simulink library "libsb2sl"  (Simulink 7.3)
settings: Solver=ode45  SolverMode=SingleTasking  StartTime=0.0  StopTime=10.0  RelTol=1e-3
PostLoadFcn:
  | setsysloc libsb2sl
undefined symbols (not defined in the file): A, Ac, Ad, B, Bc, Bd, C, Cc, Cd, code, const, D, data, Dc, Dd, DiscIntNeverNeededParam, gain, info, k, m, map, no, stat, X0, xd, xi
libraries: simulink3 x17, simulink x5, libsb2sl x3
(part 2 of 3)

== system libsb2sl/DYN/DResetIntegrator ==
  1stOrder : Subsystem  mask(DYN-Palette){IMODE=Forward Euler, RMODE=Single edge, K=1, X0=0, TS=0.1}
      mask prompts: IMODE "Integrator Method:"; RMODE "External Reset:"; K "Output Gains:"; X0 "Initial Conditions:"; TS "Sampling Time:"
      mask help: Nth order integration of an input with resettable states.
      mask init:
      | operator={'rising','either'};
      | method={'ForwardEuler';'BackwardEuler';'Trapezoidal'};
      | set_param([gcb  '/Integrator'],'ExternalReset',operator{RMODE},'IntegratorMethod',method{IMODE});
      | [x,y]=sblibico('1stOrderReset','disc');
      mask StyleString: popup(Forward Euler|Backward Euler|Trapezoidal),popup(Single edge|Double edge),edit,edit,edit
      mask Display: plot(0,0,1,1,x,y)
  1stOrder1 : Subsystem  mask(DYN-Palette){IMODE=Forward Euler, RMODE=Single edge, X0=0, TS=0.1}
      mask prompts: IMODE "Integrator Method:"; RMODE "External Reset:"; X0 "Initial Conditions:"; TS "Sampling Time:"
      mask help: Nth order integration of an input with resettable states.
      mask init:
      | operator={'rising','either'};
      | method={'ForwardEuler';'BackwardEuler';'Trapezoidal'};
      | set_param([gcb  '/Integrator'],'ExternalReset',operator{RMODE},'IntegratorMethod',method{IMODE});
      | [x,y]=sblibico('1stOrder1Reset','disc');
      mask StyleString: popup(Forward Euler|Backward Euler|Trapezoidal),popup(Single edge|Double edge),edit,edit
      mask Display: plot(0,0,1,1,x,y)
  NthOrder : Subsystem  mask(DYN-Palette){IMODE=Forward Euler, N=1, RMODE=Single edge, NR=1, K=1, X0=0, TS=0.1}
      mask prompts: IMODE "Integrator Method:"; N "Order of Integration:"; RMODE "External Reset:"; NR "Highest Order of Resettable State:"; K "Output Gains:"; X0 "Initial Conditions:"; TS "Sampling Time:"
      mask help: Nth order integration of an input with resettable states.
      mask init:
      | no=length(K);
      | [stateMap,resetMap]=sblibdrv('Integrator',N,no,NR);
      | operator={'rising','either'};
      | method={'ForwardEuler';'BackwardEuler';'Trapezoidal'};
      | set_param([gcb  '/Integrator'],'ExternalReset',operator{RMODE},'IntegratorMethod',method{IMODE});
      | [x,y]=sblibico('nthOrderReset','disc');
      mask StyleString: popup(Forward Euler|Backward Euler|Trapezoidal),edit,popup(Single edge|Double edge),edit,edit,edit,edit
      mask Display: plot(0,0,1,1,x,y)
  NthOrder1 : Subsystem  mask(DYN-Palette){IMODE=Forward Euler, N=1, RMODE=Single edge, NR=1, X0=0, TS=0.1}
      mask prompts: IMODE "Integrator Method:"; N "Order of Integration:"; RMODE "External Reset:"; NR "Highest Order of Resettable State:"; X0 "Initial Conditions:"; TS "Sampling Time:"
      mask help: Nth order integration of an input with resettable states.
      mask init:
      | no=length(X0)/N;
      | [stateMap,resetMap]=sblibdrv('Integrator',N,no,NR);
      | operator={'rising','either'};
      | method={'ForwardEuler';'BackwardEuler';'Trapezoidal'};
      | set_param([gcb  '/Integrator'],'ExternalReset',operator{RMODE},'IntegratorMethod',method{IMODE});
      | [x,y]=sblibico('nthOrder1Reset','disc');
      mask StyleString: popup(Forward Euler|Backward Euler|Trapezoidal),edit,popup(Single edge|Double edge),edit,edit,edit
      mask Display: plot(0,0,1,1,x,y)

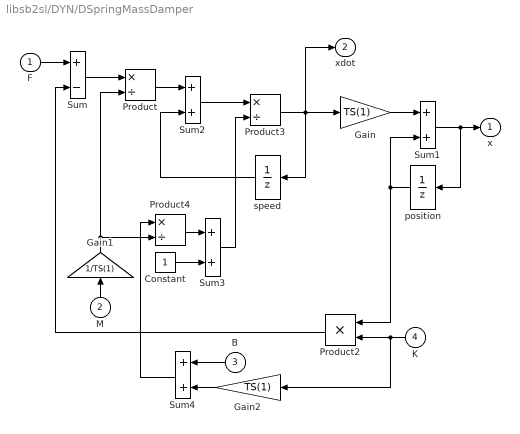
== system libsb2sl/DYN/DSpringMassDamper ==
  F : Inport  SampleTime=TS  OutDataType=sfix(16)  OutScaling=2^0
  M : Inport  Port=2  SampleTime=TS  OutDataType=sfix(16)  OutScaling=2^0
  B : Inport  Port=3  SampleTime=TS  OutDataType=sfix(16)  OutScaling=2^0
  K : Inport  Port=4  SampleTime=TS  OutDataType=sfix(16)  OutScaling=2^0
  Constant : Constant  OutDataType=sfix(16)  OutScaling=2^0
  Gain : Gain  Gain=TS(1)  ParameterDataType=sfix(16)  ParameterScaling=2^0  OutDataType=sfix(16)  OutScaling=2^0  SaturateOnIntegerOverflow=on  OutDataTypeStr=Inherit: Same as input  ParamDataTypeStr=Inherit: Same as input
  Gain1 : Gain  Gain=1/TS(1)  ParameterDataType=sfix(16)  ParameterScaling=2^0  OutDataType=sfix(16)  OutScaling=2^0  SaturateOnIntegerOverflow=on  OutDataTypeStr=Inherit: Same as input  ParamDataTypeStr=Inherit: Same as input
  Gain2 : Gain  Gain=TS(1)  ParameterDataType=sfix(16)  ParameterScaling=2^0  OutDataType=sfix(16)  OutScaling=2^0  SaturateOnIntegerOverflow=on  OutDataTypeStr=Inherit: Same as input  ParamDataTypeStr=Inherit: Same as input
  Product : Product  Inputs=*/  OutDataType=sfix(16)  OutScaling=2^0  SaturateOnIntegerOverflow=on  RndMeth=Zero  InputSameDT=on  OutDataTypeStr=Inherit: Same as first input
  Product2 : Product  OutDataType=sfix(16)  OutScaling=2^0  SaturateOnIntegerOverflow=on  RndMeth=Zero  InputSameDT=on  OutDataTypeStr=Inherit: Same as first input
  Product3 : Product  Inputs=*/  OutDataType=sfix(16)  OutScaling=2^0  SaturateOnIntegerOverflow=on  RndMeth=Zero  InputSameDT=on  OutDataTypeStr=Inherit: Same as first input
  Product4 : Product  Inputs=*/  OutDataType=sfix(16)  OutScaling=2^0  SaturateOnIntegerOverflow=on  RndMeth=Zero  InputSameDT=on  OutDataTypeStr=Inherit: Same as first input
  Sum : Sum  Inputs=+-  OutDataType=sfix(16)  OutScaling=2^0  SaturateOnIntegerOverflow=on  InputSameDT=on  OutDataTypeStr=Inherit: Same as first input
  Sum{1..4} (4 alike) : Sum  OutDataType=sfix(16)  OutScaling=2^0  SaturateOnIntegerOverflow=on  InputSameDT=on  OutDataTypeStr=Inherit: Same as first input
  position : UnitDelay  X0=X0(1)  SampleTime=TS
  speed : UnitDelay  X0=X0(2)  SampleTime=TS
  x : Outport  OutDataType=sfix(16)  OutScaling=2^0  InitialOutput=X0(1)
  xdot : Outport  Port=2  OutDataType=sfix(16)  OutScaling=2^0  InitialOutput=X0(2)
  wires:
  Sum4/1 -> Product4/1
  Gain2/1 -> Sum4/2
  B/1 -> Sum4/1
  K/1 -> Gain2/1, Product2/2
  Gain1/1 -> Product4/2, Product/2
  M/1 -> Gain1/1
  position/1 -> Product2/1, Sum1/2
  Sum3/1 -> Product3/2
  Product2/1 -> Sum/2
  Sum1/1 -> position/1, x/1
  Gain/1 -> Sum1/1
  Product3/1 -> xdot/1, Gain/1, speed/1
  Product4/1 -> Sum3/1
  Constant/1 -> Sum3/2
  speed/1 -> Sum2/2
  Sum2/1 -> Product3/1
  Product/1 -> Sum2/1
  Sum/1 -> Product/1
  F/1 -> Sum/1

== system libsb2sl/DYN/DStateSpace ==
  u : Inport  OutDataType=sfix(16)  OutScaling=2^0
  StateSpace : DiscreteStateSpace  A=A  B=B  C=C  D=D  X0=X0  SampleTime=TS
  y : Outport  OutDataType=sfix(16)  OutScaling=2^0
  wires:
  u/1 -> StateSpace/1
  StateSpace/1 -> y/1

== system libsb2sl/DYN/DTimeDelay ==
  u : Inport  SampleTime=TS  OutDataType=sfix(16)  OutScaling=2^0
  Demux : Demux  Outputs=[no no (k+1)*no]
  Mux : Mux  Inputs=[no (k+1)*no]
  Selector : Selector  InputPortWidth=(k+2)*no  IndexOptions=Index vector (dialog)  Indices=[k*no+1:(k+2)*no 1:(k+1)*no]  OutputSizes=1
  Sum : Sum  Inputs=+|+  OutDataType=sfix(16)  OutScaling=2^0  SaturateOnIntegerOverflow=on  InputSameDT=on  OutDataTypeStr=Inherit: Same as first input
  Unit Delay : UnitDelay  X0=X0  SampleTime=TS
  m : Gain  Gain=1-m  ParameterDataType=sfix(16)  ParameterScaling=2^0  OutDataType=sfix(16)  OutScaling=2^0  SaturateOnIntegerOverflow=on  OutDataTypeStr=Inherit: Same as input  ParamDataTypeStr=Inherit: Same as input
  m1 : Gain  Gain=m  ParameterDataType=sfix(16)  ParameterScaling=2^0  OutDataType=sfix(16)  OutScaling=2^0  SaturateOnIntegerOverflow=on  OutDataTypeStr=Inherit: Same as input  ParamDataTypeStr=Inherit: Same as input
  y : Outport  OutDataType=sfix(16)  OutScaling=2^0
  wires:
  u/1 -> Mux/1
  Unit Delay/1 -> Mux/2
  Mux/1 -> Selector/1
  Sum/1 -> y/1
  m1/1 -> Sum/2
  m/1 -> Sum/1
  Demux/2 -> m1/1
  Demux/1 -> m/1
  Demux/3 -> Unit Delay/1
  Selector/1 -> Demux/1

== system libsb2sl/LOG/Decoder ==
  u : Inport  OutDataType=sfix(16)  OutScaling=2^0
  decoder : S-Function  FunctionName=sbdecoder  Parameters=BPI,MIN,MAX  EnableBusSupport=off
  y : Outport  OutDataType=sfix(16)  OutScaling=2^0
  wires:
  u/1 -> decoder/1
  decoder/1 -> y/1

== system libsb2sl/LOG/EQV ==
  u1 : Inport  OutDataType=sfix(16)  OutScaling=2^0
  u2 : Inport  Port=2  OutDataType=sfix(16)  OutScaling=2^0
  EQV : Logic  Operator=NOT  Inputs=1
  NEQV : Logic  Operator=XOR
  bool1 : RelationalOperator  Operator=>  InputSameDT=on
  bool2 : RelationalOperator  Operator=>  InputSameDT=on
  zero : Constant  Value=0  OutDataType=sfix(16)  OutScaling=2^0  OutDataTypeStr=Inherit: Inherit via back propagation
  y : Outport  OutDataType=sfix(16)  OutScaling=2^0
  wires:
  bool1/1 -> NEQV/1
  bool2/1 -> NEQV/2
  u1/1 -> bool1/1
  u2/1 -> bool2/1
  zero/1 -> bool2/2, bool1/2
  NEQV/1 -> EQV/1
  EQV/1 -> y/1

== system libsb2sl/LOG/Encoder ==
  u : Inport  OutDataType=sfix(16)  OutScaling=2^0
  encoder : S-Function  FunctionName=sbencoder  Parameters=BPO,MIN,MAX  EnableBusSupport=off
  y : Outport  OutDataType=sfix(16)  OutScaling=2^0
  wires:
  u/1 -> encoder/1
  encoder/1 -> y/1

== system libsb2sl/LOG/GainScheduler ==
  s : Inport  OutDataType=sfix(16)  OutScaling=2^0
  u : Inport  Port=2  OutDataType=sfix(16)  OutScaling=2^0
  sbgainsched : S-Function  FunctionName=sbgainsched  Parameters=IND,GAIN  EnableBusSupport=off
  y : Outport  OutDataType=sfix(16)  OutScaling=2^0
  wires:
  s/1 -> sbgainsched/1
  sbgainsched/1 -> y/1
  u/1 -> sbgainsched/2

== system libsb2sl/LOG/LogExpression ==
  u : Inport  OutDataType=sfix(16)  OutScaling=2^0
  sblogexp : S-Function  FunctionName=sblogexp  Parameters=code,stat,data,info,P0,TS  EnableBusSupport=off
  y : Outport  OutDataType=sfix(16)  OutScaling=2^0
  wires:
  u/1 -> sblogexp/1
  sblogexp/1 -> y/1

== system libsb2sl/LOG/NEQV ==
  u1 : Inport  OutDataType=sfix(16)  OutScaling=2^0
  u2 : Inport  Port=2  OutDataType=sfix(16)  OutScaling=2^0
  NEQV : Logic  Operator=XOR
  bool1 : RelationalOperator  Operator=>  InputSameDT=on
  bool2 : RelationalOperator  Operator=>  InputSameDT=on
  zero : Constant  Value=0  OutDataType=sfix(16)  OutScaling=2^0  OutDataTypeStr=Inherit: Inherit via back propagation
  y : Outport  OutDataType=sfix(16)  OutScaling=2^0
  wires:
  bool1/1 -> NEQV/1
  bool2/1 -> NEQV/2
  u1/1 -> bool1/1
  NEQV/1 -> y/1
  u2/1 -> bool2/1
  zero/1 -> bool1/2, bool2/2

== system libsb2sl/LOG/NOT ==
  u1 : Inport  OutDataType=sfix(16)  OutScaling=2^0
  bool1 : RelationalOperator  Operator=>  InputSameDT=on
  logic : Logic  Operator=NOT
  zero : Constant  Value=0  OutDataType=sfix(16)  OutScaling=2^0  OutDataTypeStr=Inherit: Inherit via back propagation
  y : Outport  OutDataType=sfix(16)  OutScaling=2^0
  wires:
  bool1/1 -> logic/1
  u1/1 -> bool1/1
  logic/1 -> y/1
  zero/1 -> bool1/2

== system libsb2sl/LOG/ShiftRegister ==
  u : Inport  SampleTime=TS  OutDataType=sfix(16)  OutScaling=2^0
  sbshiftreg : S-Function  FunctionName=sbshiftreg  Parameters=NX,NY,X0,TS  EnableBusSupport=off
  y : Outport  OutDataType=sfix(16)  OutScaling=2^0
  wires:
  u/1 -> sbshiftreg/1
  sbshiftreg/1 -> y/1

== system libsb2sl/LOG/Switch ==
  u1 : Inport  OutDataType=sfix(16)  OutScaling=2^0
  u2 : Inport  Port=2  OutDataType=sfix(16)  OutScaling=2^0
  u3 : Inport  Port=3  OutDataType=sfix(16)  OutScaling=2^0
  Switch : Switch  Criteria=u2 > Threshold  SaturateOnIntegerOverflow=on  InputSameDT=on
  y : Outport  OutDataType=sfix(16)  OutScaling=2^0
  wires:
  Switch/1 -> y/1
  u2/1 -> Switch/1
  u3/1 -> Switch/3
  u1/1 -> Switch/2

== system libsb2sl/MAT/Constant ==
  Constant : Constant  Value=constantValue  OutDataType=sfix(16)  OutScaling=2^0
  Y : Outport  OutDataType=sfix(16)  OutScaling=2^0
  wires:
  Constant/1 -> Y/1

== system libsb2sl/MAT/LeftMultiply ==
  A : Inport  OutDataType=sfix(16)  OutScaling=2^0
  Matrix Gain : Gain  Gain=G  Multiplication=Matrix(u*K)  ParameterDataType=sfix(16)  ParameterScaling=2^0  OutDataType=sfix(16)  OutScaling=2^0  SaturateOnIntegerOverflow=on  OutDataTypeStr=Inherit: Same as input  ParamDataTypeStr=Inherit: Same as input
  Y2y : simulink/Math Operations/Reshape  OutputDimensionality=1-D array  OutputDimensions=[1,1]
  a2A : simulink/Math Operations/Reshape  OutputDimensionality=Customize  OutputDimensions=[nACols,nARows]
  Y : Outport  OutDataType=sfix(16)  OutScaling=2^0
  wires:
  A/1 -> a2A/1
  Y2y/1 -> Y/1
  Matrix Gain/1 -> Y2y/1
  a2A/1 -> Matrix Gain/1

== system libsb2sl/MAT/MatLeftDivide ==
  A : Inport  OutDataType=sfix(16)  OutScaling=2^0
  B : Inport  Port=2  OutDataType=sfix(16)  OutScaling=2^0
  Product : Product  Inputs=*/  Multiplication=Matrix(*)  OutDataType=sfix(16)  OutScaling=2^0  SaturateOnIntegerOverflow=on  RndMeth=Zero  InputSameDT=on  OutDataTypeStr=Inherit: Same as first input
  Y2y : simulink3/Signals & Systems/Reshape  OutputDimensionality=1-D array  OutputDimensions=[1,1]
  a2A : simulink3/Signals & Systems/Reshape  OutputDimensionality=Customize  OutputDimensions=[nACols,nARows]
  b2B : simulink3/Signals & Systems/Reshape  OutputDimensionality=Customize  OutputDimensions=[nBCols,nBRows]
  Y : Outport  OutDataType=sfix(16)  OutScaling=2^0
  wires:
  Product/1 -> Y2y/1
  B/1 -> b2B/1
  Y2y/1 -> Y/1
  A/1 -> a2A/1
  b2B/1 -> Product/1
  a2A/1 -> Product/2

== system libsb2sl/MAT/MatRightDivide ==
  A : Inport  OutDataType=sfix(16)  OutScaling=2^0
  B : Inport  Port=2  OutDataType=sfix(16)  OutScaling=2^0
  Product : Product  Inputs=/*  Multiplication=Matrix(*)  OutDataType=sfix(16)  OutScaling=2^0  SaturateOnIntegerOverflow=on  RndMeth=Zero  InputSameDT=on  OutDataTypeStr=Inherit: Same as first input
  Y2y : simulink3/Signals & Systems/Reshape  OutputDimensionality=1-D array  OutputDimensions=[1,1]
  a2A : simulink3/Signals & Systems/Reshape  OutputDimensionality=Customize  OutputDimensions=[nACols,nARows]
  b2B : simulink3/Signals & Systems/Reshape  OutputDimensionality=Customize  OutputDimensions=[nBCols,nBRows]
  Y : Outport  OutDataType=sfix(16)  OutScaling=2^0
  wires:
  b2B/1 -> Product/2
  a2A/1 -> Product/1
  Product/1 -> Y2y/1
  A/1 -> a2A/1
  Y2y/1 -> Y/1
  B/1 -> b2B/1

== system libsb2sl/MAT/MatrixInverse ==
  A : Inport  OutDataType=sfix(16)  OutScaling=2^0
  Product : Product  Inputs=/  Multiplication=Matrix(*)  OutDataType=sfix(16)  OutScaling=2^0  SaturateOnIntegerOverflow=on  RndMeth=Zero  InputSameDT=on  OutDataTypeStr=Inherit: Same as first input
  Y2y : simulink3/Signals & Systems/Reshape  OutputDimensionality=1-D array  OutputDimensions=[1,1]
  a2A : simulink3/Signals & Systems/Reshape  OutputDimensionality=Customize  OutputDimensions=[nACols,nARows]
  Y : Outport  OutDataType=sfix(16)  OutScaling=2^0
  wires:
  A/1 -> a2A/1
  Y2y/1 -> Y/1
  a2A/1 -> Product/1
  Product/1 -> Y2y/1

== system libsb2sl/MAT/MatrixMultiply ==
  A : Inport  OutDataType=sfix(16)  OutScaling=2^0
  B : Inport  Port=2  OutDataType=sfix(16)  OutScaling=2^0
  Product : Product  Inputs=**  Multiplication=Matrix(*)  OutDataType=sfix(16)  OutScaling=2^0  SaturateOnIntegerOverflow=on  RndMeth=Zero  InputSameDT=on  OutDataTypeStr=Inherit: Same as first input
  Y2y : simulink3/Signals & Systems/Reshape  OutputDimensionality=1-D array  OutputDimensions=[1,1]
  a2A : simulink3/Signals & Systems/Reshape  OutputDimensionality=Customize  OutputDimensions=[nACols,nARows]
  b2B : simulink3/Signals & Systems/Reshape  OutputDimensionality=Customize  OutputDimensions=[nBCols,nBRows]
  Y : Outport  OutDataType=sfix(16)  OutScaling=2^0
  wires:
  a2A/1 -> Product/2
  b2B/1 -> Product/1
  B/1 -> b2B/1
  Y2y/1 -> Y/1
  A/1 -> a2A/1
  Product/1 -> Y2y/1

== system libsb2sl/MAT/MatrixTranspose ==
  A : Inport  OutDataType=sfix(16)  OutScaling=2^0
  Selector : Selector  InputPortWidth=nARows*nACols  IndexOptions=Index vector (dialog)  Indices=mapIndices(:)  OutputSizes=1
  Y : Outport  OutDataType=sfix(16)  OutScaling=2^0
  wires:
  Selector/1 -> Y/1
  A/1 -> Selector/1

== system libsb2sl/MAT/RightMultiply ==
  A : Inport  OutDataType=sfix(16)  OutScaling=2^0
  Matrix Gain : Gain  Gain=G  Multiplication=Matrix(K*u)  ParameterDataType=sfix(16)  ParameterScaling=2^0  OutDataType=sfix(16)  OutScaling=2^0  SaturateOnIntegerOverflow=on  OutDataTypeStr=Inherit: Same as input  ParamDataTypeStr=Inherit: Same as input
  Y2y : Reshape
  a2A : Reshape  OutputDimensionality=Customize  OutputDimensions=[nACols,nARows]
  Y : Outport  OutDataType=sfix(16)  OutScaling=2^0
  wires:
  a2A/1 -> Matrix Gain/1
  Matrix Gain/1 -> Y2y/1
  Y2y/1 -> Y/1
  A/1 -> a2A/1

== system libsb2sl/NTP/BiCubicInterp ==
  note: Swap inputs to accommodate
      | Row-major 2-D tables in
      | SystemBuild
  u1 : Inport  OutDataType=sfix(16)  OutScaling=2^0
  u2 : Inport  Port=2  OutDataType=sfix(16)  OutScaling=2^0
  Look-Up Table (n-D) : simulink3/Functions & Tables/Look-Up Table (n-D)  numDimsPopupSelect=2  bp1=in2BrkPoints  bp2=in1BrkPoints  explicitNumDims=2  searchMode=Binary Search  cacheBpFlag=on  vectorInputFlag=off  tableData=outBrkPoints  interpMethod=Cubic Spline  extrapMethod=None - Clip  rangeErrorMode=Error
  y : Outport  OutDataType=sfix(16)  OutScaling=2^0
  wires:
  u1/1 -> Look-Up Table (n-D)/2
  u2/1 -> Look-Up Table (n-D)/1
  Look-Up Table (n-D)/1 -> y/1

== system libsb2sl/NTP/BiLinearInterp ==
  note: Swap inputs to accommodate
      | Row-major 2-D tables in
      | SystemBuild
  u1 : Inport  OutDataType=sfix(16)  OutScaling=2^0
  u2 : Inport  Port=2  OutDataType=sfix(16)  OutScaling=2^0
  Look-Up Table (n-D) : simulink3/Functions & Tables/Look-Up Table (n-D)  numDimsPopupSelect=2  bp1=in2BrkPoints  bp2=in1BrkPoints  explicitNumDims=2  searchMode=Binary Search  cacheBpFlag=on  vectorInputFlag=off  tableData=outBrkPoints  interpMethod=Linear  extrapMethod=Linear  rangeErrorMode=None
  y : Outport  OutDataType=sfix(16)  OutScaling=2^0
  wires:
  u2/1 -> Look-Up Table (n-D)/1
  u1/1 -> Look-Up Table (n-D)/2
  Look-Up Table (n-D)/1 -> y/1

== system libsb2sl/NTP/ConstantInterp ==
  u : Inport  OutDataType=sfix(16)  OutScaling=2^0
  Look-Up Table (n-D) : simulink3/Functions & Tables/Look-Up Table (n-D)  numDimsPopupSelect=1  bp1=in1BrkPoints  explicitNumDims=1  searchMode=Binary Search  cacheBpFlag=on  vectorInputFlag=on  tableData=outBrkPoints  interpMethod=None - Flat  extrapMethod=None - Clip  rangeErrorMode=None
  y : Outport  OutDataType=sfix(16)  OutScaling=2^0
  wires:
  Look-Up Table (n-D)/1 -> y/1
  u/1 -> Look-Up Table (n-D)/1

== system libsb2sl/NTP/CubicInterp ==
  u : Inport  OutDataType=sfix(16)  OutScaling=2^0
  Look-Up Table (n-D) : simulink3/Functions & Tables/Look-Up Table (n-D)  numDimsPopupSelect=1  bp1=in1BrkPoints  explicitNumDims=1  searchMode=Binary Search  cacheBpFlag=on  vectorInputFlag=on  tableData=outBrkPoints  interpMethod=Cubic Spline  extrapMethod=Cubic Spline  rangeErrorMode=None
  y : Outport  OutDataType=sfix(16)  OutScaling=2^0
  wires:
  u/1 -> Look-Up Table (n-D)/1
  Look-Up Table (n-D)/1 -> y/1

== system libsb2sl/NTP/LinearInterp ==
  u : Inport  OutDataType=sfix(16)  OutScaling=2^0
  Look-Up Table (n-D) : simulink3/Functions & Tables/Look-Up Table (n-D)  numDimsPopupSelect=1  bp1=in1BrkPoints  explicitNumDims=1  searchMode=Binary Search  cacheBpFlag=on  vectorInputFlag=on  tableData=outBrkPoints  interpMethod=Linear  extrapMethod=Linear  rangeErrorMode=None
  y : Outport  OutDataType=sfix(16)  OutScaling=2^0
  wires:
  u/1 -> Look-Up Table (n-D)/1
  Look-Up Table (n-D)/1 -> y/1

== system libsb2sl/NTP/MultiLinearInterp ==
  u : Inport  OutDataType=sfix(16)  OutScaling=2^0
  multilinear interp : simulink/Lookup Tables/Lookup Table (n-D)  numDimsPopupSelect=More...  bp1=in1BrkPoints  bp2=in2BrkPoints  bp3=in3BrkPoints  bp4=in4BrkPoints  bpcell={in5BrkPoints,in6BrkPoints,in7BrkPoints,in8BrkPoints}  explicitNumDims=NINP+1  searchMode=Linear Search  cacheBpFlag=on  vectorInputFlag=on  tableData=tableData  interpMethod=Linear  extrapMethod=Linear  rangeErrorMode=None
  y : Outport  OutDataType=sfix(16)  OutScaling=2^0
  wires:
  multilinear interp/1 -> y/1
  u/1 -> multilinear interp/1

== system libsb2sl/PEL/Constant**u ==
  u : Inport  OutDataType=sfix(16)  OutScaling=2^0
  Constant : Constant  Value=CONST  OutDataType=sfix(16)  OutScaling=2^0
  Power : Math  Operator=pow  OutDataType=sfix(16)  OutScaling=2^0  SaturateOnIntegerOverflow=on
  y : Outport  OutDataType=sfix(16)  OutScaling=2^0
  wires:
  Power/1 -> y/1
  Constant/1 -> Power/1
  u/1 -> Power/2

== system libsb2sl/PEL/SignedSqrt ==
  u : Inport  OutDataType=sfix(16)  OutScaling=2^0
  Abs : Abs  SaturateOnIntegerOverflow=on
  Math Function : Math  Operator=sqrt  OutDataType=sfix(16)  OutScaling=2^0  SaturateOnIntegerOverflow=on
  Product : Product  OutDataType=sfix(16)  OutScaling=2^0  SaturateOnIntegerOverflow=on  RndMeth=Zero  InputSameDT=on  OutDataTypeStr=Inherit: Same as first input
  Sign : Signum
  y : Outport  OutDataType=sfix(16)  OutScaling=2^0
  wires:
  Math Function/1 -> Product/1
  Sign/1 -> Product/2
  Abs/1 -> Math Function/1
  Product/1 -> y/1
  u/1 -> Abs/1, Sign/1

== system libsb2sl/PEL/u**Constant ==
  u : Inport  OutDataType=sfix(16)  OutScaling=2^0
  Constant : Constant  Value=CONST  OutDataType=sfix(16)  OutScaling=2^0
  Power : Math  Operator=pow  OutDataType=sfix(16)  OutScaling=2^0  SaturateOnIntegerOverflow=on
  y : Outport  OutDataType=sfix(16)  OutScaling=2^0
  wires:
  Power/1 -> y/1
  u/1 -> Power/1
  Constant/1 -> Power/2

== system libsb2sl/PWL/Preload ==
  u : Inport  OutDataType=sfix(16)  OutScaling=2^0
  Constant : Constant  Value=preload  OutDataType=sfix(16)  OutScaling=2^0
  Constant1 : Constant  Value=-preload  OutDataType=sfix(16)  OutScaling=2^0
  Sum : Sum  OutDataType=sfix(16)  OutScaling=2^0  SaturateOnIntegerOverflow=on  InputSameDT=on  OutDataTypeStr=Inherit: Same as first input
  Switch : Switch  SaturateOnIntegerOverflow=on  InputSameDT=on
  slope : Gain  Gain=slope  ParameterDataType=sfix(16)  ParameterScaling=2^0  OutDataType=sfix(16)  OutScaling=2^0  SaturateOnIntegerOverflow=on  OutDataTypeStr=Inherit: Same as input  ParamDataTypeStr=Inherit: Same as input
  y : Outport  OutDataType=sfix(16)  OutScaling=2^0
  wires:
  slope/1 -> Sum/2
  Switch/1 -> Sum/1
  u/1 -> Switch/2, slope/1
  Sum/1 -> y/1
  Constant/1 -> Switch/1
  Constant1/1 -> Switch/3

== system libsb2sl/PWL/Quantization ==
  u : Inport  OutDataType=sfix(16)  OutScaling=2^0
  Resolution : Constant  Value=RES  OutDataType=sfix(16)  OutScaling=2^0
  Type : Rounding  Operator=round
  div : Product  Inputs=*/  OutDataType=sfix(16)  OutScaling=2^0  SaturateOnIntegerOverflow=on  RndMeth=Zero  InputSameDT=on  OutDataTypeStr=Inherit: Same as first input
  mul : Product  OutDataType=sfix(16)  OutScaling=2^0  SaturateOnIntegerOverflow=on  RndMeth=Zero  InputSameDT=on  OutDataTypeStr=Inherit: Same as first input
  y : Outport  OutDataType=sfix(16)  OutScaling=2^0
  wires:
  div/1 -> Type/1
  Type/1 -> mul/1
  Resolution/1 -> div/2, mul/2
  u/1 -> div/1
  mul/1 -> y/1

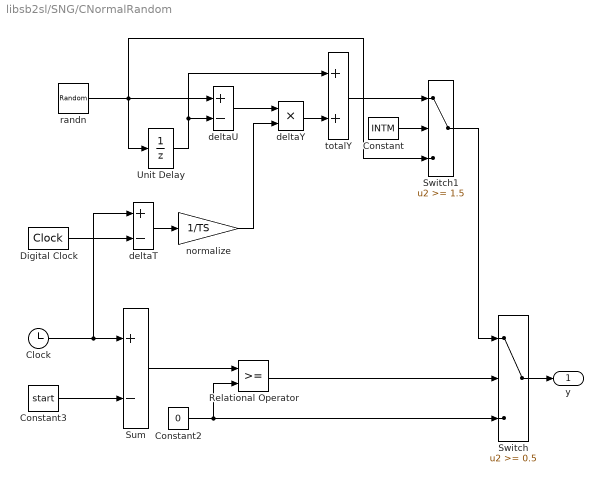
== system libsb2sl/SNG/CNormalRandom ==
  Clock : Clock
      settings: Decimation=10
  Constant : Constant  Value=INTM  OutDataType=sfix(16)  OutScaling=2^0
  Constant2 : Constant  Value=0  OutDataType=sfix(16)  OutScaling=2^0
  Constant3 : Constant  Value=start  OutDataType=sfix(16)  OutScaling=2^0
  Digital Clock : DigitalClock  SampleTime=TS
  Relational Operator : RelationalOperator  InputSameDT=on
  Sum : Sum  Inputs=+-  OutDataType=sfix(16)  OutScaling=2^0  SaturateOnIntegerOverflow=on  InputSameDT=on  OutDataTypeStr=Inherit: Same as first input
  Switch : Switch  Threshold=0.5  SaturateOnIntegerOverflow=on  InputSameDT=on
  Switch1 : Switch  Threshold=1.5  SaturateOnIntegerOverflow=on  InputSameDT=on
  Unit Delay : UnitDelay  SampleTime=TS
  deltaT : Sum  Inputs=+-  OutDataType=sfix(16)  OutScaling=2^0  SaturateOnIntegerOverflow=on  InputSameDT=on  OutDataTypeStr=Inherit: Same as first input
  deltaU : Sum  Inputs=+-  OutDataType=sfix(16)  OutScaling=2^0  SaturateOnIntegerOverflow=on  InputSameDT=on  OutDataTypeStr=Inherit: Same as first input
  deltaY : Product  OutDataType=sfix(16)  OutScaling=2^0  SaturateOnIntegerOverflow=on  RndMeth=Zero  InputSameDT=on  OutDataTypeStr=Inherit: Same as first input
  normalize : Gain  Gain=1/TS  ParameterDataType=sfix(16)  ParameterScaling=2^0  OutDataType=sfix(16)  OutScaling=2^0  SaturateOnIntegerOverflow=on  OutDataTypeStr=Inherit: Same as input  ParamDataTypeStr=Inherit: Same as input
  randn : RandomNumber  Mean=MEAN  Variance=STD.^2  Seed=SEED  SampleTime=TS
  totalY : Sum  OutDataType=sfix(16)  OutScaling=2^0  SaturateOnIntegerOverflow=on  InputSameDT=on  OutDataTypeStr=Inherit: Same as first input
  y : Outport  OutDataType=sfix(16)  OutScaling=2^0
  wires:
  Clock/1 -> deltaT/1, Sum/1
  Switch/1 -> y/1
  Switch1/1 -> Switch/1
  Constant2/1 -> Switch/3, Relational Operator/2
  Relational Operator/1 -> Switch/2
  Sum/1 -> Relational Operator/1
  Constant3/1 -> Sum/2
  randn/1 -> deltaU/1, Unit Delay/1, Switch1/3
  Constant/1 -> Switch1/2
  totalY/1 -> Switch1/1
  Unit Delay/1 -> deltaU/2, totalY/1
  deltaY/1 -> totalY/2
  normalize/1 -> deltaY/2
  deltaU/1 -> deltaY/1
  deltaT/1 -> normalize/1
  Digital Clock/1 -> deltaT/2

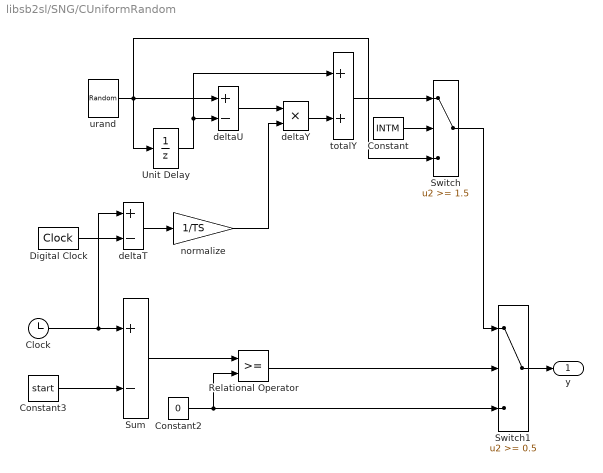
== system libsb2sl/SNG/CUniformRandom ==
  Clock : Clock
      settings: Decimation=10
  Constant : Constant  Value=INTM  OutDataType=sfix(16)  OutScaling=2^0
  Constant2 : Constant  Value=0  OutDataType=sfix(16)  OutScaling=2^0
  Constant3 : Constant  Value=start  OutDataType=sfix(16)  OutScaling=2^0
  Digital Clock : DigitalClock  SampleTime=TS
  Relational Operator : RelationalOperator  InputSameDT=on
  Sum : Sum  Inputs=+-  OutDataType=sfix(16)  OutScaling=2^0  SaturateOnIntegerOverflow=on  InputSameDT=on  OutDataTypeStr=Inherit: Same as first input
  Switch : Switch  Threshold=1.5  SaturateOnIntegerOverflow=on  InputSameDT=on
  Switch1 : Switch  Threshold=0.5  SaturateOnIntegerOverflow=on  InputSameDT=on
  Unit Delay : UnitDelay  SampleTime=TS
  deltaT : Sum  Inputs=+-  OutDataType=sfix(16)  OutScaling=2^0  SaturateOnIntegerOverflow=on  InputSameDT=on  OutDataTypeStr=Inherit: Same as first input
  deltaU : Sum  Inputs=+-  OutDataType=sfix(16)  OutScaling=2^0  SaturateOnIntegerOverflow=on  InputSameDT=on  OutDataTypeStr=Inherit: Same as first input
  deltaY : Product  OutDataType=sfix(16)  OutScaling=2^0  SaturateOnIntegerOverflow=on  RndMeth=Zero  InputSameDT=on  OutDataTypeStr=Inherit: Same as first input
  normalize : Gain  Gain=1/TS  ParameterDataType=sfix(16)  ParameterScaling=2^0  OutDataType=sfix(16)  OutScaling=2^0  SaturateOnIntegerOverflow=on  OutDataTypeStr=Inherit: Same as input  ParamDataTypeStr=Inherit: Same as input
  totalY : Sum  OutDataType=sfix(16)  OutScaling=2^0  SaturateOnIntegerOverflow=on  InputSameDT=on  OutDataTypeStr=Inherit: Same as first input
  urand : UniformRandomNumber  Minimum=MIN  Maximum=MAX  Seed=SEED  SampleTime=TS
  y : Outport  OutDataType=sfix(16)  OutScaling=2^0
  wires:
  Constant2/1 -> Relational Operator/2, Switch1/3
  Relational Operator/1 -> Switch1/2
  Sum/1 -> Relational Operator/1
  Constant3/1 -> Sum/2
  Switch1/1 -> y/1
  Constant/1 -> Switch/2
  totalY/1 -> Switch/1
  Unit Delay/1 -> totalY/1, deltaU/2
  deltaY/1 -> totalY/2
  normalize/1 -> deltaY/2
  deltaU/1 -> deltaY/1
  deltaT/1 -> normalize/1
  Digital Clock/1 -> deltaT/2
  urand/1 -> Switch/3, Unit Delay/1, deltaU/1
  Switch/1 -> Switch1/1
  Clock/1 -> Sum/1, deltaT/1

== system libsb2sl/SNG/DNormalRandom ==
  Clock : Clock
      settings: Decimation=10
  Constant2 : Constant  Value=0  OutDataType=sfix(16)  OutScaling=2^0
  Constant3 : Constant  Value=start  OutDataType=sfix(16)  OutScaling=2^0
  Relational Operator : RelationalOperator  InputSameDT=on
  Sum : Sum  Inputs=+-  OutDataType=sfix(16)  OutScaling=2^0  SaturateOnIntegerOverflow=on  InputSameDT=on  OutDataTypeStr=Inherit: Same as first input
  Switch : Switch  Threshold=0.5  SaturateOnIntegerOverflow=on  InputSameDT=on
  randn : RandomNumber  Mean=MEAN  Variance=STD.^2  Seed=SEED  SampleTime=TS
  y : Outport  OutDataType=sfix(16)  OutScaling=2^0
  wires:
  randn/1 -> Switch/1
  Clock/1 -> Sum/1
  Constant3/1 -> Sum/2
  Sum/1 -> Relational Operator/1
  Relational Operator/1 -> Switch/2
  Constant2/1 -> Relational Operator/2, Switch/3
  Switch/1 -> y/1

== system libsb2sl/SNG/DUniformRandom ==
  Clock : Clock
      settings: Decimation=10
  Constant2 : Constant  Value=0  OutDataType=sfix(16)  OutScaling=2^0
  Constant3 : Constant  Value=start  OutDataType=sfix(16)  OutScaling=2^0
  Relational Operator : RelationalOperator  InputSameDT=on
  Sum : Sum  Inputs=+-  OutDataType=sfix(16)  OutScaling=2^0  SaturateOnIntegerOverflow=on  InputSameDT=on  OutDataTypeStr=Inherit: Same as first input
  Switch : Switch  Threshold=0.5  SaturateOnIntegerOverflow=on  InputSameDT=on
  urand : UniformRandomNumber  Minimum=MIN  Maximum=MAX  Seed=SEED  SampleTime=TS
  y : Outport  OutDataType=sfix(16)  OutScaling=2^0
  wires:
  Clock/1 -> Sum/1
  Constant3/1 -> Sum/2
  Sum/1 -> Relational Operator/1
  Relational Operator/1 -> Switch/2
  Constant2/1 -> Switch/3, Relational Operator/2
  Switch/1 -> y/1
  urand/1 -> Switch/1

== system libsb2sl/SNG/GenWaveform ==
  Clock : Clock
      settings: Decimation=10
  Constant1 : Constant  Value=period  OutDataType=sfix(16)  OutScaling=2^0
  Constant2 : Constant  Value=0  OutDataType=sfix(16)  OutScaling=2^0
  Constant3 : Constant  Value=start  OutDataType=sfix(16)  OutScaling=2^0
  LinearInterp : libsb2sl/NTP/LinearInterp  SystemSampleTime=-1  in1BrkPoints=in1BrkPoints  outBrkPoints=outBrkPoints
  Math Function : Math  Operator=rem  OutDataType=sfix(16)  OutScaling=2^0  SaturateOnIntegerOverflow=on
  Sum : Sum  Inputs=+-  OutDataType=sfix(16)  OutScaling=2^0  SaturateOnIntegerOverflow=on  InputSameDT=on  OutDataTypeStr=Inherit: Same as first input
  Switch : Switch  SaturateOnIntegerOverflow=on  InputSameDT=on
  y : Outport  OutDataType=sfix(16)  OutScaling=2^0
  wires:
  Clock/1 -> Sum/1
  Switch/1 -> y/1
  Sum/1 -> Math Function/1, Switch/2
  Constant3/1 -> Sum/2
  Constant2/1 -> Switch/3
  Constant1/1 -> Math Function/2
  Math Function/1 -> LinearInterp/1
  LinearInterp/1 -> Switch/1

== system libsb2sl/SNG/LimRamp ==
  Compare To Zero : simulink/Logic and Bit Operations/Compare To Zero  SystemSampleTime=-1  relop=~=  LogicOutDataTypeMode=boolean  ZeroCross=off
  Constant5 : Constant  Value=SAT  OutDataType=sfix(16)  OutScaling=2^0
  Constant6 : Constant  Value=RATE  OutDataType=sfix(16)  OutScaling=2^0
  Data Type Conversion : DataTypeConversion  OutDataType=fixdt(1, 16)  OutScaling=2^0
  Product : Product  OutDataType=sfix(16)  OutScaling=2^0  SaturateOnIntegerOverflow=on  RndMeth=Zero  InputSameDT=on  OutDataTypeStr=Inherit: Same as first input
  Product1 : Product  OutDataType=sfix(16)  OutScaling=2^0  SaturateOnIntegerOverflow=on  RndMeth=Zero  InputSameDT=on  OutDataTypeStr=Inherit: Same as first input
  Ramp : simulink/Sources/Ramp  SystemSampleTime=-1  slope=RATE  start=start  X0=0
  Sum1 : Sum  Inputs=-+  OutDataType=sfix(16)  OutScaling=2^0  SaturateOnIntegerOverflow=on  InputSameDT=on  OutDataTypeStr=Inherit: Same as first input
  Switch1 : Switch  SaturateOnIntegerOverflow=on  InputSameDT=on
  y : Outport  OutDataType=sfix(16)  OutScaling=2^0
  wires:
  Data Type Conversion/1 -> Product1/2
  Product1/1 -> Switch1/3
  Compare To Zero/1 -> Data Type Conversion/1
  Ramp/1 -> Compare To Zero/1, Switch1/1, Sum1/1
  Constant6/1 -> Product/2
  Sum1/1 -> Product/1
  Constant5/1 -> Product1/1, Sum1/2
  Switch1/1 -> y/1
  Product/1 -> Switch1/2

== system libsb2sl/SNG/PulseTrain ==
  Pulse Generator1 : DiscretePulseGenerator  PulseType=Time based  Amplitude=A  Period=1./F  PulseWidth=PW.*F*100  PhaseDelay=start  SampleTime=1
  y : Outport  OutDataType=sfix(16)  OutScaling=2^0
  wires:
  Pulse Generator1/1 -> y/1

== system libsb2sl/SNG/SinusoidGen ==
  Clock : Clock
      settings: Decimation=10
  Constant2 : Constant  Value=0  OutDataType=sfix(16)  OutScaling=2^0
  Constant3 : Constant  Value=start  OutDataType=sfix(16)  OutScaling=2^0
  Relational Operator : RelationalOperator  InputSameDT=on
  Sine Wave : Sin  TimeSource=Use external signal  Amplitude=A  Bias=0  Frequency=2*pi*F  Phase=pi*PHI/180  Samples=10  SampleTime=0  Offset=0
  Sum : Sum  Inputs=+-  OutDataType=sfix(16)  OutScaling=2^0  SaturateOnIntegerOverflow=on  InputSameDT=on  OutDataTypeStr=Inherit: Same as first input
  Switch : Switch  Threshold=0.5  SaturateOnIntegerOverflow=on  InputSameDT=on
  y : Outport  OutDataType=sfix(16)  OutScaling=2^0
  wires:
  Switch/1 -> y/1
  Sine Wave/1 -> Switch/1
  Constant2/1 -> Switch/3, Relational Operator/2
  Relational Operator/1 -> Switch/2
  Constant3/1 -> Sum/2
  Clock/1 -> Sum/1
  Sum/1 -> Sine Wave/1, Relational Operator/1

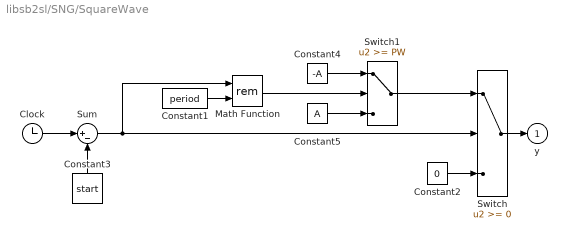
== system libsb2sl/SNG/SquareWave ==
  Clock : Clock
      settings: Decimation=10
  Constant1 : Constant  Value=period  OutDataType=sfix(16)  OutScaling=2^0
  Constant2 : Constant  Value=0  OutDataType=sfix(16)  OutScaling=2^0
  Constant3 : Constant  Value=start  OutDataType=sfix(16)  OutScaling=2^0
  Constant4 : Constant  Value=-A  OutDataType=sfix(16)  OutScaling=2^0
  Constant5 : Constant  Value=A  OutDataType=sfix(16)  OutScaling=2^0
  Math Function : Math  Operator=rem  OutDataType=sfix(16)  OutScaling=2^0  SaturateOnIntegerOverflow=on
  Sum : Sum  Inputs=|+-  OutDataType=sfix(16)  OutScaling=2^0  SaturateOnIntegerOverflow=on  InputSameDT=on  OutDataTypeStr=Inherit: Same as first input
  Switch : Switch  SaturateOnIntegerOverflow=on  InputSameDT=on
  Switch1 : Switch  Threshold=PW  SaturateOnIntegerOverflow=on  InputSameDT=on
  y : Outport  OutDataType=sfix(16)  OutScaling=2^0
  wires:
  Constant5/1 -> Switch1/3
  Constant4/1 -> Switch1/1
  Switch1/1 -> Switch/1
  Math Function/1 -> Switch1/2
  Switch/1 -> y/1
  Constant3/1 -> Sum/2
  Sum/1 -> Math Function/1, Switch/2
  Clock/1 -> Sum/1
  Constant2/1 -> Switch/3
  Constant1/1 -> Math Function/2

== system libsb2sl/SNG/StepFcn ==
  Step : Step  Time=start  After=A  SampleTime=TS
  y : Outport  OutDataType=sfix(16)  OutScaling=2^0
  wires:
  Step/1 -> y/1

== system libsb2sl/SUP/DataStoreRW ==
  u : Inport  PortDimensions=NREG  SampleTime=TS  OutDataType=sfix(16)  OutScaling=2^0
  Mux : Mux  Inputs=2
  Selector : Selector  InputPortWidth=inpWidth  IndexOptions=Index vector (dialog)  Indices=inputMap  OutputSizes=1
  dsRead : DataStoreRead  Priority=1  DataStoreName=VAR  SampleTime=TS
  dsWrite : DataStoreWrite  Priority=2  DataStoreName=VAR  SampleTime=TS
  y : Outport  OutDataType=sfix(16)  OutScaling=2^0
  wires:
  u/1 -> Mux/1
  Mux/1 -> Selector/1
  dsRead/1 -> Mux/2
  Selector/1 -> dsWrite/1, y/1

== system libsb2sl/SUP/DataStoreW ==
  u : Inport  PortDimensions=NREG  SampleTime=TS  OutDataType=sfix(16)  OutScaling=2^0
  Mux : Mux  Inputs=2
  Selector : Selector  InputPortWidth=inpWidth  IndexOptions=Index vector (dialog)  Indices=inputMap  OutputSizes=1
  dsRead : DataStoreRead  Priority=1  DataStoreName=VAR  SampleTime=TS
  dsWrite : DataStoreWrite  Priority=2  DataStoreName=VAR  SampleTime=TS
  wires:
  Mux/1 -> Selector/1
  u/1 -> Mux/1
  Selector/1 -> dsWrite/1
  dsRead/1 -> Mux/2

== system libsb2sl/TRG/CosAsin ==
  u : Inport  OutDataType=sfix(16)  OutScaling=2^0
  asin : Trigonometry  Operator=asin
  cos : Trigonometry  Operator=cos
  y : Outport  OutDataType=sfix(16)  OutScaling=2^0
  wires:
  cos/1 -> y/1
  u/1 -> asin/1
  asin/1 -> cos/1

== system libsb2sl/TRG/CosAtan2 ==
  u1 : Inport  OutDataType=sfix(16)  OutScaling=2^0
  u2 : Inport  Port=2  OutDataType=sfix(16)  OutScaling=2^0
  atan2 : Trigonometry  Operator=atan2
  cosine : Trigonometry  Operator=cos
  y : Outport  OutDataType=sfix(16)  OutScaling=2^0
  wires:
  cosine/1 -> y/1
  atan2/1 -> cosine/1
  u2/1 -> atan2/2
  u1/1 -> atan2/1

== system libsb2sl/TRG/SinAtan2 ==
  u1 : Inport  OutDataType=sfix(16)  OutScaling=2^0
  u2 : Inport  Port=2  OutDataType=sfix(16)  OutScaling=2^0
  arctangent2 : Trigonometry  Operator=atan2
  sine : Trigonometry
  y : Outport  OutDataType=sfix(16)  OutScaling=2^0
  wires:
  u2/1 -> arctangent2/2
  sine/1 -> y/1
  u1/1 -> arctangent2/1
  arctangent2/1 -> sine/1

== system libsb2sl/USR/BlockScript ==
  u : Inport  OutDataType=sfix(16)  OutScaling=2^0
  BlockScriptCode : S-Function  FunctionName=foo  Parameters=SIZES,X0  EnableBusSupport=off
  y : Outport  OutDataType=sfix(16)  OutScaling=2^0
  wires:
  BlockScriptCode/1 -> y/1
  u/1 -> BlockScriptCode/1

== system libsb2sl/USR/ZIBlockScript ==
  BlockScriptCode : S-Function  FunctionName=foo  Parameters=SIZES,X0  EnableBusSupport=off
  Ground : Ground
  y : Outport  OutDataType=sfix(16)  OutScaling=2^0
  wires:
  BlockScriptCode/1 -> y/1
  Ground/1 -> BlockScriptCode/1

== system libsb2sl/ALG/AlgExpression/Constant ==
  Constant : Constant  Value=const  OutDataType=sfix(16)  OutScaling=2^0
  y : Outport  OutDataType=sfix(16)  OutScaling=2^0
  wires:
  Constant/1 -> y/1

== system libsb2sl/ALG/AlgExpression/Offset ==
  u : Inport  OutDataType=sfix(16)  OutScaling=2^0
  Constant : Constant  Value=const  OutDataType=sfix(16)  OutScaling=2^0
  Gain : Gain  Gain=sign  ParameterDataType=sfix(16)  ParameterScaling=2^0  OutDataType=sfix(16)  OutScaling=2^0  SaturateOnIntegerOverflow=on  OutDataTypeStr=Inherit: Same as input  ParamDataTypeStr=Inherit: Same as input
  Selector : Selector  InputPortWidth=ni  IndexOptions=Index vector (dialog)  Indices=map  OutputSizes=1
  Sum : Sum  Inputs=|++  OutDataType=sfix(16)  OutScaling=2^0  SaturateOnIntegerOverflow=on  InputSameDT=on  OutDataTypeStr=Inherit: Same as first input
  y : Outport  OutDataType=sfix(16)  OutScaling=2^0
  wires:
  Constant/1 -> Sum/1
  Gain/1 -> Sum/2
  Sum/1 -> y/1
  Selector/1 -> Gain/1
  u/1 -> Selector/1

== system libsb2sl/ALG/AlgExpression/PowerCU ==
  u : Inport  OutDataType=sfix(16)  OutScaling=2^0
  Constant : Constant  Value=const  OutDataType=sfix(16)  OutScaling=2^0
  Gain : Gain  Gain=sign  ParameterDataType=sfix(16)  ParameterScaling=2^0  OutDataType=sfix(16)  OutScaling=2^0  SaturateOnIntegerOverflow=on  OutDataTypeStr=Inherit: Same as input  ParamDataTypeStr=Inherit: Same as input
  Math Function : Math  Operator=pow  OutDataType=sfix(16)  OutScaling=2^0  SaturateOnIntegerOverflow=on
  Selector : Selector  InputPortWidth=ni  IndexOptions=Index vector (dialog)  Indices=map  OutputSizes=1
  y : Outport  OutDataType=sfix(16)  OutScaling=2^0
  wires:
  Math Function/1 -> Gain/1
  Gain/1 -> y/1
  Constant/1 -> Math Function/1
  u/1 -> Selector/1
  Selector/1 -> Math Function/2

== system libsb2sl/ALG/AlgExpression/Product ==
  u : Inport  OutDataType=sfix(16)  OutScaling=2^0
  Gain : Gain  Gain=sign  ParameterDataType=sfix(16)  ParameterScaling=2^0  OutDataType=sfix(16)  OutScaling=2^0  SaturateOnIntegerOverflow=on  OutDataTypeStr=Inherit: Same as input  ParamDataTypeStr=Inherit: Same as input
  Product : Product  Inputs=**  OutDataType=sfix(16)  OutScaling=2^0  SaturateOnIntegerOverflow=on  RndMeth=Zero  InputSameDT=on  OutDataTypeStr=Inherit: Same as first input
  Selector : Selector  InputPortWidth=ni  IndexOptions=Index vector (dialog)  Indices=map(:,1)  OutputSizes=1
  Selector1 : Selector  InputPortWidth=ni  IndexOptions=Index vector (dialog)  Indices=map(:,2)  OutputSizes=1
  y : Outport  OutDataType=sfix(16)  OutScaling=2^0
  wires:
  Gain/1 -> y/1
  Product/1 -> Gain/1
  u/1 -> Selector/1, Selector1/1
  Selector/1 -> Product/1
  Selector1/1 -> Product/2

== system libsb2sl/ALG/AlgExpression/Reciprocal ==
  u : Inport  OutDataType=sfix(16)  OutScaling=2^0
  Constant : Constant  Value=const  OutDataType=sfix(16)  OutScaling=2^0
  Div : Product  Inputs=*/  OutDataType=sfix(16)  OutScaling=2^0  SaturateOnIntegerOverflow=on  RndMeth=Zero  InputSameDT=on  OutDataTypeStr=Inherit: Same as first input
  Selector : Selector  InputPortWidth=ni  IndexOptions=Index vector (dialog)  Indices=map  OutputSizes=1
  y : Outport  OutDataType=sfix(16)  OutScaling=2^0
  wires:
  u/1 -> Selector/1
  Selector/1 -> Div/2
  Constant/1 -> Div/1
  Div/1 -> y/1

== system libsb2sl/ALG/AlgExpression/Scale ==
  u : Inport  OutDataType=sfix(16)  OutScaling=2^0
  Gain : Gain  Gain=gain  ParameterDataType=sfix(16)  ParameterScaling=2^0  OutDataType=sfix(16)  OutScaling=2^0  SaturateOnIntegerOverflow=on  OutDataTypeStr=Inherit: Same as input  ParamDataTypeStr=Inherit: Same as input
  Selector : Selector  InputPortWidth=ni  IndexOptions=Index vector (dialog)  Indices=map  OutputSizes=1
  y : Outport  OutDataType=sfix(16)  OutScaling=2^0
  wires:
  Gain/1 -> y/1
  Selector/1 -> Gain/1
  u/1 -> Selector/1

== system libsb2sl/ALG/AlgExpression/Summation ==
  u : Inport  OutDataType=sfix(16)  OutScaling=2^0
  Gain : Gain  Gain=sign(:,1)  ParameterDataType=sfix(16)  ParameterScaling=2^0  OutDataType=sfix(16)  OutScaling=2^0  SaturateOnIntegerOverflow=on  OutDataTypeStr=Inherit: Same as input  ParamDataTypeStr=Inherit: Same as input
  Gain1 : Gain  Gain=sign(:,2)  ParameterDataType=sfix(16)  ParameterScaling=2^0  OutDataType=sfix(16)  OutScaling=2^0  SaturateOnIntegerOverflow=on  OutDataTypeStr=Inherit: Same as input  ParamDataTypeStr=Inherit: Same as input
  Selector : Selector  InputPortWidth=ni  IndexOptions=Index vector (dialog)  Indices=map(:,1)  OutputSizes=1
  Selector1 : Selector  InputPortWidth=ni  IndexOptions=Index vector (dialog)  Indices=map(:,2)  OutputSizes=1
  Sum : Sum  Inputs=|++  OutDataType=sfix(16)  OutScaling=2^0  SaturateOnIntegerOverflow=on  InputSameDT=on  OutDataTypeStr=Inherit: Same as first input
  y : Outport  OutDataType=sfix(16)  OutScaling=2^0
  wires:
  Sum/1 -> y/1
  u/1 -> Selector1/1, Selector/1
  Gain1/1 -> Sum/2
  Selector1/1 -> Gain1/1
  Gain/1 -> Sum/1
  Selector/1 -> Gain/1

== system libsb2sl/DYN/CIntegrator/1stOrder ==
  u : Inport  OutDataType=sfix(16)  OutScaling=2^0
  Gain : Gain  Gain=K  ParameterDataType=sfix(16)  ParameterScaling=2^0  OutDataType=sfix(16)  OutScaling=2^0  SaturateOnIntegerOverflow=on  OutDataTypeStr=Inherit: Same as input  ParamDataTypeStr=Inherit: Same as input
  Integrator : Integrator  InitialCondition=X0
  y : Outport  OutDataType=sfix(16)  OutScaling=2^0
  wires:
  Gain/1 -> y/1
  u/1 -> Integrator/1
  Integrator/1 -> Gain/1

== system libsb2sl/DYN/CIntegrator/NthOrder ==
  u : Inport  OutDataType=sfix(16)  OutScaling=2^0
  Demux : Demux  Outputs=[no no*N]
  Gain : Gain  Gain=K  ParameterDataType=sfix(16)  ParameterScaling=2^0  OutDataType=sfix(16)  OutScaling=2^0  SaturateOnIntegerOverflow=on  OutDataTypeStr=Inherit: Same as input  ParamDataTypeStr=Inherit: Same as input
  Integrator : Integrator  InitialCondition=X0
  Mux : Mux  Inputs=[no no*N]
  StateMap : Selector  InputPortWidth=no*(1+N)  IndexOptions=Index vector (dialog)  Indices=stateMap  OutputSizes=1
  y : Outport  OutDataType=sfix(16)  OutScaling=2^0
  wires:
  Gain/1 -> y/1
  Demux/1 -> Gain/1
  u/1 -> Mux/1
  Demux/2 -> Integrator/1
  Integrator/1 -> Mux/2
  StateMap/1 -> Demux/1
  Mux/1 -> StateMap/1

== system libsb2sl/DYN/CIntegrator/NthOrder1 ==
  u : Inport  OutDataType=sfix(16)  OutScaling=2^0
  Demux : Demux  Outputs=[no no*N]
  Integrator : Integrator  InitialCondition=X0
  Mux : Mux  Inputs=[no no*N]
  StateMap : Selector  InputPortWidth=no*(1+N)  IndexOptions=Index vector (dialog)  Indices=stateMap  OutputSizes=1
  y : Outport  OutDataType=sfix(16)  OutScaling=2^0
  wires:
  Mux/1 -> StateMap/1
  StateMap/1 -> Demux/1
  Integrator/1 -> Mux/2
  Demux/2 -> Integrator/1
  u/1 -> Mux/1
  Demux/1 -> y/1

== system libsb2sl/DYN/CPIDControlLaw/D Term ==
  e : Inport  OutDataType=sfix(16)  OutScaling=2^0
  Enable D Term : EnablePort  StatesWhenEnabling=reset
  Derivative : Gain  Gain=D  ParameterDataType=sfix(16)  ParameterScaling=2^0  OutDataType=sfix(16)  OutScaling=2^0  SaturateOnIntegerOverflow=on  OutDataTypeStr=Inherit: Same as input  ParamDataTypeStr=Inherit: Same as input
  Sum1 : Sum  Inputs=|+-  OutDataType=sfix(16)  OutScaling=2^0  SaturateOnIntegerOverflow=on  InputSameDT=on  OutDataTypeStr=Inherit: Same as first input
  TimeConstant : Gain  Gain=1/TAU  ParameterDataType=sfix(16)  ParameterScaling=2^0  OutDataType=sfix(16)  OutScaling=2^0  SaturateOnIntegerOverflow=on  OutDataTypeStr=Inherit: Same as input  ParamDataTypeStr=Inherit: Same as input
  xd : Integrator  InitialCondition=xd
  u_d : Outport  OutDataType=sfix(16)  OutScaling=2^0
  wires:
  e/1 -> Sum1/1
  xd/1 -> Sum1/2
  TimeConstant/1 -> xd/1, Derivative/1
  Sum1/1 -> TimeConstant/1
  Derivative/1 -> u_d/1

== system libsb2sl/DYN/CPIDControlLaw/I Term ==
  e : Inport  OutDataType=sfix(16)  OutScaling=2^0
  Enable I Term : EnablePort  StatesWhenEnabling=reset
  Integral : Gain  Gain=I  ParameterDataType=sfix(16)  ParameterScaling=2^0  OutDataType=sfix(16)  OutScaling=2^0  SaturateOnIntegerOverflow=on  OutDataTypeStr=Inherit: Same as input  ParamDataTypeStr=Inherit: Same as input
  xi : Integrator  InitialCondition=xi
  u_i : Outport  OutDataType=sfix(16)  OutScaling=2^0
  wires:
  e/1 -> xi/1
  xi/1 -> Integral/1
  Integral/1 -> u_i/1

== system libsb2sl/DYN/CResetIntegrator/1stOrder ==
  u : Inport  OutDataType=sfix(16)  OutScaling=2^0
  new : Inport  Port=2  OutDataType=sfix(16)  OutScaling=2^0
  reset : Inport  Port=3  OutDataType=sfix(16)  OutScaling=2^0
  Gain : Gain  Gain=K  ParameterDataType=sfix(16)  ParameterScaling=2^0  OutDataType=sfix(16)  OutScaling=2^0  SaturateOnIntegerOverflow=on  OutDataTypeStr=Inherit: Same as input  ParamDataTypeStr=Inherit: Same as input
  IC : InitialCondition  Value=X0
  Integrator : Integrator  ExternalReset=rising  InitialConditionSource=external  InitialCondition=X0
  y : Outport  OutDataType=sfix(16)  OutScaling=2^0
  wires:
  reset/1 -> Integrator/2
  IC/1 -> Integrator/3
  new/1 -> IC/1
  u/1 -> Integrator/1
  Integrator/1 -> Gain/1
  Gain/1 -> y/1

== system libsb2sl/DYN/CResetIntegrator/1stOrder1 ==
  u : Inport  OutDataType=sfix(16)  OutScaling=2^0
  new : Inport  Port=2  OutDataType=sfix(16)  OutScaling=2^0
  reset : Inport  Port=3  OutDataType=sfix(16)  OutScaling=2^0
  IC : InitialCondition  Value=X0
  Integrator : Integrator  ExternalReset=rising  InitialConditionSource=external  InitialCondition=X0
  y : Outport  OutDataType=sfix(16)  OutScaling=2^0
  wires:
  Integrator/1 -> y/1
  u/1 -> Integrator/1
  new/1 -> IC/1
  IC/1 -> Integrator/3
  reset/1 -> Integrator/2

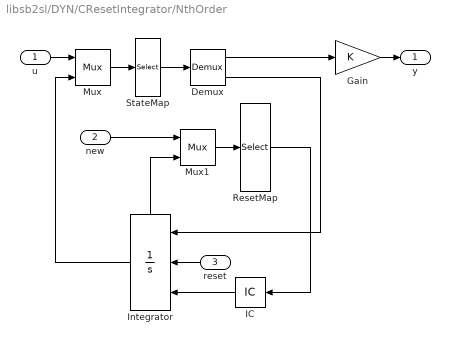
== system libsb2sl/DYN/CResetIntegrator/NthOrder ==
  u : Inport  OutDataType=sfix(16)  OutScaling=2^0
  new : Inport  Port=2  OutDataType=sfix(16)  OutScaling=2^0
  reset : Inport  Port=3  OutDataType=sfix(16)  OutScaling=2^0
  Demux : Demux  Outputs=[no no*N]
  Gain : Gain  Gain=K  ParameterDataType=sfix(16)  ParameterScaling=2^0  OutDataType=sfix(16)  OutScaling=2^0  SaturateOnIntegerOverflow=on  OutDataTypeStr=Inherit: Same as input  ParamDataTypeStr=Inherit: Same as input
  IC : InitialCondition  Value=X0
  Integrator : Integrator  ExternalReset=rising  InitialConditionSource=external  InitialCondition=X0  ShowStatePort=on
  Mux : Mux  Inputs=[no no*N]
  Mux1 : Mux  Inputs=[NR N]*no
  ResetMap : Selector  InputPortWidth=(NR+N)*no  IndexOptions=Index vector (dialog)  Indices=resetMap  OutputSizes=1
  StateMap : Selector  InputPortWidth=no*(1+N)  IndexOptions=Index vector (dialog)  Indices=stateMap  OutputSizes=1
  y : Outport  OutDataType=sfix(16)  OutScaling=2^0
  wires:
  Demux/1 -> Gain/1
  u/1 -> Mux/1
  StateMap/1 -> Demux/1
  Mux/1 -> StateMap/1
  IC/1 -> Integrator/3
  Integrator/1 -> Mux/2
  reset/1 -> Integrator/2
  ResetMap/1 -> IC/1
  new/1 -> Mux1/1
  Mux1/1 -> ResetMap/1
  Integrator/State -> Mux1/2
  Gain/1 -> y/1
  Demux/2 -> Integrator/1

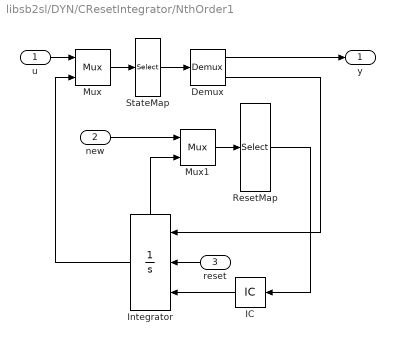
== system libsb2sl/DYN/CResetIntegrator/NthOrder1 ==
  u : Inport  OutDataType=sfix(16)  OutScaling=2^0
  new : Inport  Port=2  OutDataType=sfix(16)  OutScaling=2^0
  reset : Inport  Port=3  OutDataType=sfix(16)  OutScaling=2^0
  Demux : Demux  Outputs=[no no*N]
  IC : InitialCondition  Value=X0
  Integrator : Integrator  ExternalReset=rising  InitialConditionSource=external  InitialCondition=X0  ShowStatePort=on
  Mux : Mux  Inputs=[no no*N]
  Mux1 : Mux  Inputs=[NR N]*no
  ResetMap : Selector  InputPortWidth=(NR+N)*no  IndexOptions=Index vector (dialog)  Indices=resetMap  OutputSizes=1
  StateMap : Selector  InputPortWidth=no*(1+N)  IndexOptions=Index vector (dialog)  Indices=stateMap  OutputSizes=1
  y : Outport  OutDataType=sfix(16)  OutScaling=2^0
  wires:
  Demux/2 -> Integrator/1
  Integrator/State -> Mux1/2
  Mux1/1 -> ResetMap/1
  new/1 -> Mux1/1
  ResetMap/1 -> IC/1
  reset/1 -> Integrator/2
  Integrator/1 -> Mux/2
  IC/1 -> Integrator/3
  Mux/1 -> StateMap/1
  StateMap/1 -> Demux/1
  u/1 -> Mux/1
  Demux/1 -> y/1

== system libsb2sl/DYN/DIntegrator/1stOrder ==
  u : Inport  SampleTime=TS  OutDataType=sfix(16)  OutScaling=2^0
  Gain : Gain  Gain=K  ParameterDataType=sfix(16)  ParameterScaling=2^0  OutDataType=sfix(16)  OutScaling=2^0  SaturateOnIntegerOverflow=on  OutDataTypeStr=Inherit: Same as input  ParamDataTypeStr=Inherit: Same as input
  Integrator : DiscreteIntegrator  InitialCondition=X0  SampleTime=TS  OutDataType=sfix(16)  OutScaling=2^0  ICPrevOutput=DiscIntNeverNeededParam  ICPrevScaledInput=DiscIntNeverNeededParam
  y : Outport  OutDataType=sfix(16)  OutScaling=2^0
  wires:
  u/1 -> Integrator/1
  Gain/1 -> y/1
  Integrator/1 -> Gain/1
